simulink model "pipeline_13bit"  (R2022b)
settings: Solver=FixedStepDiscrete  StartTime=0.0  StopTime=5000*ts  FixedStep=ts  RelTol=1e-3
values from neighbouring files (symbols this model uses):
  beta = 1.01    [ADC_13bit.m]
  bits_number = 13    [ADC_13bit.m]
  C = 10e-12    (= 1e-11)    [ADC_13bit.m]
  fin = antismear(fin_pre,fs,nfft)    [ADC_13bit.m]
  Gain = 5000    [ADC_13bit.m]
  k = 1.380649e-23    [ADC_13bit.m]
  T = 300    [ADC_13bit.m]
  ts = 1/fs    (= 1)    [ADC_13bit.m]
(part 2 of 3)

== system pipeline_13bit/SHA_less_13_bit/Adder/Add6 ==
  A : Inport
  B : Inport  Port=2
  C : Inport  Port=3
  Combinatorial Logic1 : CombinatorialLogic  TruthTable=[0 0;1 0 ;1 0;0 1;1 0;0 1;0 1;1 1]
  Data Type Conversion : DataTypeConversion  OutDataTypeStr=boolean  SaturateOnIntegerOverflow=off  RndMeth=Floor
  Data Type Conversion1 : DataTypeConversion  OutDataTypeStr=double  SaturateOnIntegerOverflow=off  RndMeth=Floor
  Demux : Demux  Outputs=2
  Mux : Mux  Inputs=3
  Carry : Outport
  Sum : Outport  Port=2
  wires:
  Demux/1 -> Sum/1
  Demux/2 -> Carry/1
  Combinatorial Logic1/1 -> Data Type Conversion1/1
  Mux/1 -> Data Type Conversion/1
  A/1 -> Mux/3
  B/1 -> Mux/2
  C/1 -> Mux/1
  Data Type Conversion1/1 -> Demux/1
  Data Type Conversion/1 -> Combinatorial Logic1/1

== system pipeline_13bit/SHA_less_13_bit/Adder/Add7 ==
  A : Inport
  B : Inport  Port=2
  C : Inport  Port=3
  Combinatorial Logic1 : CombinatorialLogic  TruthTable=[0 0;1 0 ;1 0;0 1;1 0;0 1;0 1;1 1]
  Data Type Conversion : DataTypeConversion  OutDataTypeStr=boolean  SaturateOnIntegerOverflow=off  RndMeth=Floor
  Data Type Conversion1 : DataTypeConversion  OutDataTypeStr=double  SaturateOnIntegerOverflow=off  RndMeth=Floor
  Demux : Demux  Outputs=2
  Mux : Mux  Inputs=3
  Carry : Outport
  Sum : Outport  Port=2
  wires:
  Demux/1 -> Sum/1
  Demux/2 -> Carry/1
  Combinatorial Logic1/1 -> Data Type Conversion1/1
  Mux/1 -> Data Type Conversion/1
  A/1 -> Mux/3
  B/1 -> Mux/2
  C/1 -> Mux/1
  Data Type Conversion1/1 -> Demux/1
  Data Type Conversion/1 -> Combinatorial Logic1/1

== system pipeline_13bit/SHA_less_13_bit/Adder/Add8 ==
  A : Inport
  B : Inport  Port=2
  C : Inport  Port=3
  Combinatorial Logic1 : CombinatorialLogic  TruthTable=[0 0;1 0 ;1 0;0 1;1 0;0 1;0 1;1 1]
  Data Type Conversion : DataTypeConversion  OutDataTypeStr=boolean  SaturateOnIntegerOverflow=off  RndMeth=Floor
  Data Type Conversion1 : DataTypeConversion  OutDataTypeStr=double  SaturateOnIntegerOverflow=off  RndMeth=Floor
  Demux : Demux  Outputs=2
  Mux : Mux  Inputs=3
  Carry : Outport
  Sum : Outport  Port=2
  wires:
  Demux/1 -> Sum/1
  Demux/2 -> Carry/1
  Combinatorial Logic1/1 -> Data Type Conversion1/1
  Mux/1 -> Data Type Conversion/1
  A/1 -> Mux/3
  B/1 -> Mux/2
  C/1 -> Mux/1
  Data Type Conversion1/1 -> Demux/1
  Data Type Conversion/1 -> Combinatorial Logic1/1

== system pipeline_13bit/SHA_less_13_bit/Adder/Add9 ==
  A : Inport
  B : Inport  Port=2
  C : Inport  Port=3
  Combinatorial Logic1 : CombinatorialLogic  TruthTable=[0 0;1 0 ;1 0;0 1;1 0;0 1;0 1;1 1]
  Data Type Conversion : DataTypeConversion  OutDataTypeStr=boolean  SaturateOnIntegerOverflow=off  RndMeth=Floor
  Data Type Conversion1 : DataTypeConversion  OutDataTypeStr=double  SaturateOnIntegerOverflow=off  RndMeth=Floor
  Demux : Demux  Outputs=2
  Mux : Mux  Inputs=3
  Carry : Outport
  Sum : Outport  Port=2
  wires:
  Demux/1 -> Sum/1
  Demux/2 -> Carry/1
  Combinatorial Logic1/1 -> Data Type Conversion1/1
  Mux/1 -> Data Type Conversion/1
  A/1 -> Mux/3
  B/1 -> Mux/2
  C/1 -> Mux/1
  Data Type Conversion1/1 -> Demux/1
  Data Type Conversion/1 -> Combinatorial Logic1/1

== system pipeline_13bit/SHA_less_13_bit/Subsystem/stage_1p5_bit1 ==
  note: b2
  note: b1
  Vin : Inport
  Comparator 1 : Subsystem
  Comparator 2 : Subsystem
  Encoder : Subsystem
  Gain1 : Gain  Gain=2
  Gain2 : Gain
  Gain3 : Gain
  Saturation : Saturate  UpperLimit=1  LowerLimit=-1
  Sub DAC : Subsystem
  Subsystem1 : Subsystem
  Sum : Sum  Inputs=|+-
  Vref 1 : Constant  Value=-1/4
  Vref 2 : Constant  Value=1/4
  Zero-Order Hold : ZeroOrderHold  SampleTime=ts
  Residue : Outport
  D0 : Outport  Port=2
  D1 : Outport  Port=3
  wires:
  Vref 1/1 -> Comparator 1/2(Vref)
  Gain1/1 -> Sum/1
  Gain3/1 -> Sum/2
  Sum/1 -> Gain2/1
  Saturation/1 -> Zero-Order Hold/1
  Zero-Order Hold/1 -> Residue/1
  Gain2/1 -> Saturation/1
  Vref 2/1 -> Comparator 2/2(Vref)
  Comparator 2/1(Out) -> Sub DAC/2(b2), Encoder/2(b2)
  Vin/1 -> Subsystem1/1(IN)
  Comparator 1/1(Out) -> Encoder/1(b1), Sub DAC/1(b1)
  Subsystem1/1(S/H) -> Gain1/1, Comparator 1/1(Vin), Comparator 2/1(Vin)
  Sub DAC/1(Vdac) -> Gain3/1
  Encoder/1(D0) -> D0/1
  Encoder/2(D1) -> D1/1

== system pipeline_13bit/SHA_less_13_bit/Subsystem/stage_1p5_bit2 ==
  note: b2
  note: b1
  Vin : Inport
  Comparator 1 : Subsystem
  Comparator 2 : Subsystem
  Encoder : Subsystem
  Gain1 : Gain  Gain=2
  Gain2 : Gain
  Gain3 : Gain
  Saturation : Saturate  UpperLimit=1  LowerLimit=-1
  Sub DAC : Subsystem
  Subsystem1 : Subsystem
  Sum : Sum  Inputs=|+-
  Vref 1 : Constant  Value=-1/4
  Vref 2 : Constant  Value=1/4
  Zero-Order Hold : ZeroOrderHold  SampleTime=ts
  Residue : Outport
  D0 : Outport  Port=2
  D1 : Outport  Port=3
  wires:
  Vref 1/1 -> Comparator 1/2(Vref)
  Gain1/1 -> Sum/1
  Gain3/1 -> Sum/2
  Sum/1 -> Gain2/1
  Saturation/1 -> Zero-Order Hold/1
  Zero-Order Hold/1 -> Residue/1
  Gain2/1 -> Saturation/1
  Vref 2/1 -> Comparator 2/2(Vref)
  Comparator 2/1(Out) -> Sub DAC/2(b2), Encoder/2(b2)
  Vin/1 -> Subsystem1/1(IN)
  Comparator 1/1(Out) -> Encoder/1(b1), Sub DAC/1(b1)
  Subsystem1/1(S/H) -> Gain1/1, Comparator 1/1(Vin), Comparator 2/1(Vin)
  Sub DAC/1(Vdac) -> Gain3/1
  Encoder/1(D0) -> D0/1
  Encoder/2(D1) -> D1/1

== system pipeline_13bit/SHA_less_13_bit/Subsystem/stage_1p5_bit4 ==
  note: b2
  note: b1
  Vin : Inport
  Comparator 1 : Subsystem
  Comparator 2 : Subsystem
  Encoder : Subsystem
  Gain1 : Gain  Gain=2
  Gain2 : Gain
  Gain3 : Gain
  Saturation : Saturate  UpperLimit=1  LowerLimit=-1
  Sub DAC : Subsystem
  Subsystem1 : Subsystem
  Sum : Sum  Inputs=|+-
  Vref 1 : Constant  Value=-1/4
  Vref 2 : Constant  Value=1/4
  Zero-Order Hold : ZeroOrderHold  SampleTime=ts
  Residue : Outport
  D0 : Outport  Port=2
  D1 : Outport  Port=3
  wires:
  Vref 1/1 -> Comparator 1/2(Vref)
  Gain1/1 -> Sum/1
  Gain3/1 -> Sum/2
  Sum/1 -> Gain2/1
  Saturation/1 -> Zero-Order Hold/1
  Zero-Order Hold/1 -> Residue/1
  Gain2/1 -> Saturation/1
  Vref 2/1 -> Comparator 2/2(Vref)
  Comparator 2/1(Out) -> Sub DAC/2(b2), Encoder/2(b2)
  Vin/1 -> Subsystem1/1(IN)
  Comparator 1/1(Out) -> Encoder/1(b1), Sub DAC/1(b1)
  Subsystem1/1(S/H) -> Gain1/1, Comparator 1/1(Vin), Comparator 2/1(Vin)
  Sub DAC/1(Vdac) -> Gain3/1
  Encoder/1(D0) -> D0/1
  Encoder/2(D1) -> D1/1

== system pipeline_13bit/SHA_less_13_bit/Subsystem/stage_1p5_bit5 ==
  note: b2
  note: b1
  Vin : Inport
  Comparator 1 : Subsystem
  Comparator 2 : Subsystem
  Encoder : Subsystem
  Gain1 : Gain  Gain=2
  Gain2 : Gain
  Gain3 : Gain
  Saturation : Saturate  UpperLimit=1  LowerLimit=-1
  Sub DAC : Subsystem
  Subsystem1 : Subsystem
  Sum : Sum  Inputs=|+-
  Vref 1 : Constant  Value=-1/4
  Vref 2 : Constant  Value=1/4
  Zero-Order Hold : ZeroOrderHold  SampleTime=ts
  Residue : Outport
  D0 : Outport  Port=2
  D1 : Outport  Port=3
  wires:
  Vref 1/1 -> Comparator 1/2(Vref)
  Gain1/1 -> Sum/1
  Gain3/1 -> Sum/2
  Sum/1 -> Gain2/1
  Saturation/1 -> Zero-Order Hold/1
  Zero-Order Hold/1 -> Residue/1
  Gain2/1 -> Saturation/1
  Vref 2/1 -> Comparator 2/2(Vref)
  Comparator 2/1(Out) -> Sub DAC/2(b2), Encoder/2(b2)
  Vin/1 -> Subsystem1/1(IN)
  Comparator 1/1(Out) -> Encoder/1(b1), Sub DAC/1(b1)
  Subsystem1/1(S/H) -> Gain1/1, Comparator 1/1(Vin), Comparator 2/1(Vin)
  Sub DAC/1(Vdac) -> Gain3/1
  Encoder/1(D0) -> D0/1
  Encoder/2(D1) -> D1/1

== system pipeline_13bit/SHA_less_13_bit/Subsystem/stage_1p5_bit6 ==
  note: b2
  note: b1
  Vin : Inport
  Comparator 1 : Subsystem
  Comparator 2 : Subsystem
  Encoder : Subsystem
  Gain1 : Gain  Gain=2
  Gain2 : Gain
  Gain3 : Gain
  Saturation : Saturate  UpperLimit=1  LowerLimit=-1
  Sub DAC : Subsystem
  Subsystem1 : Subsystem
  Sum : Sum  Inputs=|+-
  Vref 1 : Constant  Value=-1/4
  Vref 2 : Constant  Value=1/4
  Zero-Order Hold : ZeroOrderHold  SampleTime=ts
  Residue : Outport
  D0 : Outport  Port=2
  D1 : Outport  Port=3
  wires:
  Vref 1/1 -> Comparator 1/2(Vref)
  Gain1/1 -> Sum/1
  Gain3/1 -> Sum/2
  Sum/1 -> Gain2/1
  Saturation/1 -> Zero-Order Hold/1
  Zero-Order Hold/1 -> Residue/1
  Gain2/1 -> Saturation/1
  Vref 2/1 -> Comparator 2/2(Vref)
  Comparator 2/1(Out) -> Sub DAC/2(b2), Encoder/2(b2)
  Vin/1 -> Subsystem1/1(IN)
  Comparator 1/1(Out) -> Encoder/1(b1), Sub DAC/1(b1)
  Subsystem1/1(S/H) -> Gain1/1, Comparator 1/1(Vin), Comparator 2/1(Vin)
  Sub DAC/1(Vdac) -> Gain3/1
  Encoder/1(D0) -> D0/1
  Encoder/2(D1) -> D1/1

== system pipeline_13bit/SHA_less_13_bit/Subsystem/stage_1p5_bit7 ==
  note: b2
  note: b1
  Vin : Inport
  Comparator 1 : Subsystem
  Comparator 2 : Subsystem
  Encoder : Subsystem
  Gain1 : Gain  Gain=2
  Gain2 : Gain
  Gain3 : Gain
  Saturation : Saturate  UpperLimit=1  LowerLimit=-1
  Sub DAC : Subsystem
  Subsystem1 : Subsystem
  Sum : Sum  Inputs=|+-
  Vref 1 : Constant  Value=-1/4
  Vref 2 : Constant  Value=1/4
  Zero-Order Hold : ZeroOrderHold  SampleTime=ts
  Residue : Outport
  D0 : Outport  Port=2
  D1 : Outport  Port=3
  wires:
  Vref 1/1 -> Comparator 1/2(Vref)
  Gain1/1 -> Sum/1
  Gain3/1 -> Sum/2
  Sum/1 -> Gain2/1
  Saturation/1 -> Zero-Order Hold/1
  Zero-Order Hold/1 -> Residue/1
  Gain2/1 -> Saturation/1
  Vref 2/1 -> Comparator 2/2(Vref)
  Comparator 2/1(Out) -> Sub DAC/2(b2), Encoder/2(b2)
  Vin/1 -> Subsystem1/1(IN)
  Comparator 1/1(Out) -> Encoder/1(b1), Sub DAC/1(b1)
  Subsystem1/1(S/H) -> Gain1/1, Comparator 1/1(Vin), Comparator 2/1(Vin)
  Sub DAC/1(Vdac) -> Gain3/1
  Encoder/1(D0) -> D0/1
  Encoder/2(D1) -> D1/1

== system pipeline_13bit/SHA_less_13_bit/Subsystem/stage_1p5_bit8 ==
  note: b2
  note: b1
  Vin : Inport
  Comparator 1 : Subsystem
  Comparator 2 : Subsystem
  Encoder : Subsystem
  Gain1 : Gain  Gain=2
  Gain2 : Gain
  Gain3 : Gain
  Saturation : Saturate  UpperLimit=1  LowerLimit=-1
  Sub DAC : Subsystem
  Subsystem1 : Subsystem
  Sum : Sum  Inputs=|+-
  Vref 1 : Constant  Value=-1/4
  Vref 2 : Constant  Value=1/4
  Zero-Order Hold : ZeroOrderHold  SampleTime=ts
  Residue : Outport
  D0 : Outport  Port=2
  D1 : Outport  Port=3
  wires:
  Vref 1/1 -> Comparator 1/2(Vref)
  Gain1/1 -> Sum/1
  Gain3/1 -> Sum/2
  Sum/1 -> Gain2/1
  Saturation/1 -> Zero-Order Hold/1
  Zero-Order Hold/1 -> Residue/1
  Gain2/1 -> Saturation/1
  Vref 2/1 -> Comparator 2/2(Vref)
  Comparator 2/1(Out) -> Sub DAC/2(b2), Encoder/2(b2)
  Vin/1 -> Subsystem1/1(IN)
  Comparator 1/1(Out) -> Encoder/1(b1), Sub DAC/1(b1)
  Subsystem1/1(S/H) -> Gain1/1, Comparator 1/1(Vin), Comparator 2/1(Vin)
  Sub DAC/1(Vdac) -> Gain3/1
  Encoder/1(D0) -> D0/1
  Encoder/2(D1) -> D1/1

== system pipeline_13bit/SHA_less_13_bit/Subsystem/stage_3_bit_flash ==
  Vin : Inport
  Comparator 1 : Subsystem
  Comparator 2 : Subsystem
  Comparator 3 : Subsystem
  Comparator 4 : Subsystem
  Comparator 5 : Subsystem
  Comparator 6 : Subsystem
  Comparator 7 : Subsystem
  Subsystem1 : Subsystem
  Thermometer to Binary Encoder : Subsystem
  Vref 1 : Constant  Value=-3/4
  Vref 2 : Constant  Value=-2/4
  Vref 3 : Constant  Value=-1/4
  Vref 4 : Constant  Value=0
  Vref 5 : Constant  Value=1/4
  Vref 6 : Constant  Value=2/4
  Vref 7 : Constant  Value=3/4
  Zero-Order Hold : ZeroOrderHold  SampleTime=ts
  D0 : Outport
  D1 : Outport  Port=2
  D2 : Outport  Port=3
  wires:
  Vin/1 -> Subsystem1/1(IN)
  Vref 1/1 -> Comparator 1/2(Vref)
  Thermometer to Binary Encoder/1(D0) -> D0/1
  Thermometer to Binary Encoder/2(D1) -> D1/1
  Thermometer to Binary Encoder/3(D2) -> D2/1
  Comparator 1/1(Out) -> Thermometer to Binary Encoder/1(b1)
  Vref 2/1 -> Comparator 2/2(Vref)
  Comparator 2/1(Out) -> Thermometer to Binary Encoder/2(b2)
  Vref 3/1 -> Comparator 3/2(Vref)
  Comparator 3/1(Out) -> Thermometer to Binary Encoder/3(b3)
  Vref 4/1 -> Comparator 4/2(Vref)
  Comparator 4/1(Out) -> Thermometer to Binary Encoder/4(b4)
  Vref 5/1 -> Comparator 5/2(Vref)
  Comparator 5/1(Out) -> Thermometer to Binary Encoder/5(b5)
  Vref 6/1 -> Comparator 6/2(Vref)
  Comparator 6/1(Out) -> Thermometer to Binary Encoder/6(b6)
  Vref 7/1 -> Comparator 7/2(Vref)
  Comparator 7/1(Out) -> Thermometer to Binary Encoder/7(b7)
  Zero-Order Hold/1 -> Comparator 1/1(Vin), Comparator 2/1(Vin), Comparator 3/1(Vin), Comparator 4/1(Vin), Comparator 5/1(Vin), Comparator 6/1(Vin), Comparator 7/1(Vin)
  Subsystem1/1(S/H) -> Zero-Order Hold/1

== system pipeline_13bit/SHA_less_13_bit/Subsystem/stage_3p5_bit ==
  Vin : Inport
  Encoder : Subsystem
  Gain1 : Gain  Gain=8
  Gain2 : Gain
  Gain3 : Gain
  Saturation : Saturate  UpperLimit=1000  LowerLimit=-1
  Sub ADC : Subsystem
      settings: PortSchema="{\"entries\":[{\"content\":{\"sides\":[{\"content\":{\"connectorIds\":[]},\"type\":\"ConnectorPlacement.EquallySpacedRectSide\",\"uuid\":\"1d580c1c-4142-4e48-88a4-e1fd0f0e227e\"},{\"content\":{\"connectorIds\":[\"Out1\",\"Out2\",\"Out3\",\"Out4\",\"Out5\",\"Out6\",\"Out7\",\"Out8\",\"Out9\",\"Out10\",\"Out11\",\"Out12\",\"Out13\",\"Out14\"],\"side\":\"RIGHT\"},\"type\":\"ConnectorPlacement.EquallySpacedRectSide\",\"uuid\":\"3d052ec1-94f1-45dc-924d-acfea8c79606\"},{\"content\":{\"connectorIds\":[\"In1\"],\"side\":\"TOP\"},\"type\":\"ConnectorPlacement.EquallySpacedRectSide\",\"uuid\":\"20df264a-1a70-4325-b402-c0ed20a64841\"}]},\"type\":\"ConnectorPlacement.EquallySpacedConnector\",\"uuid\":\"3e6ddb48-a356-47ca-8914-cd3660926421\"}],\"packageUris\":[\"http://schema.mathworks.com/mf0/Connector/R2020b\"],\"version\":\"1.0\"}"
  Sub DAC : Subsystem
      settings: PortSchema="{\"entries\":[{\"content\":{\"sides\":[{\"content\":{\"connectorIds\":[\"In1\",\"In2\",\"In3\",\"In4\",\"In5\",\"In6\",\"In7\",\"In8\",\"In9\",\"In10\",\"In11\",\"In12\",\"In13\",\"In14\"]},\"type\":\"ConnectorPlacement.EquallySpacedRectSide\",\"uuid\":\"d439bcb5-51fb-4878-814b-2d8ac36d8f53\"},{\"content\":{\"connectorIds\":[],\"side\":\"RIGHT\"},\"type\":\"ConnectorPlacement.EquallySpacedRectSide\",\"uuid\":\"a7e6c2a3-22c0-4c5a-aa3b-05f7415ac298\"},{\"content\":{\"connectorIds\":[\"Out1\"],\"side\":\"TOP\"},\"type\":\"ConnectorPlacement.EquallySpacedRectSide\",\"uuid\":\"e0a2b774-5ae1-46ea-b76d-1a34ecfd289b\"}]},\"type\":\"ConnectorPlacement.EquallySpacedConnector\",\"uuid\":\"f57b1e36-985f-4826-993f-0988339ac824\"}],\"packageUris\":[\"http://schema.mathworks.com/mf0/Connector/R2020b\"],\"version\":\"1.0\"}"
  Subsystem1 : Subsystem
  Sum : Sum  Inputs=|+-
  Zero-Order Hold : ZeroOrderHold  SampleTime=ts
  Residue : Outport
  D0 : Outport  Port=2
  D1 : Outport  Port=3
  D2 : Outport  Port=4
  D3 : Outport  Port=5
  wires:
  Gain1/1 -> Sum/1
  Gain3/1 -> Sum/2
  Sum/1 -> Gain2/1
  Saturation/1 -> Zero-Order Hold/1
  Gain2/1 -> Saturation/1
  Encoder/1(D0) -> D0/1
  Encoder/3(D2) -> D2/1
  Encoder/2(D1) -> D1/1
  Vin/1 -> Subsystem1/1(IN)
  Encoder/4(D3) -> D3/1
  Zero-Order Hold/1 -> Residue/1
  Subsystem1/1(S/H) -> Gain1/1, Sub ADC/1(Vin)
  Sub ADC/1(b1) -> Encoder/1(b1), Sub DAC/1(b1)
  Sub ADC/2(b2) -> Encoder/2(b2), Sub DAC/2(b2)
  Sub ADC/3(b3) -> Sub DAC/3(b3), Encoder/3(b3)
  Sub ADC/4(b4) -> Sub DAC/4(b4), Encoder/4(b4)
  Sub ADC/5(b5) -> Sub DAC/5(b5), Encoder/5(b5)
  Sub ADC/6(b6) -> Encoder/6(b6), Sub DAC/6(b6)
  Sub ADC/7(b7) -> Encoder/7(b7), Sub DAC/7(b7)
  Sub ADC/8(b8) -> Encoder/8(b8), Sub DAC/8(b8)
  Sub ADC/9(b9) -> Encoder/9(b9), Sub DAC/9(b9)
  Sub ADC/10(b10) -> Encoder/10(b10), Sub DAC/10(b10)
  Sub ADC/11(b11) -> Sub DAC/11(b11), Encoder/11(b11)
  Sub ADC/12(b12) -> Sub DAC/12(b12), Encoder/12(b12)
  Sub ADC/13(b13) -> Encoder/13(b13), Sub DAC/13(b13)
  Sub ADC/14(b14) -> Encoder/14(b14), Sub DAC/14(b14)
  Sub DAC/1(Vdac) -> Gain3/1

== system pipeline_13bit/13_bit/Subsystem/Subsystem/Clock Jitter ==
  IN : Inport
  Derivative : Derivative
  Product : Product
  Random Number : RandomNumber  SampleTime=ts
  Sum : Sum
  Zero-Order Hold2 : ZeroOrderHold  SampleTime=ts
  Zero-Order Hold3 : ZeroOrderHold  SampleTime=ts
  delta : Gain  Gain=0.02
  Clock : Outport
  wires:
  IN/1 -> Derivative/1, Sum/1
  Product/1 -> Sum/2
  Derivative/1 -> Product/1
  Zero-Order Hold2/1 -> delta/1
  Sum/1 -> Zero-Order Hold3/1
  delta/1 -> Product/2
  Zero-Order Hold3/1 -> Clock/1
  Random Number/1 -> Zero-Order Hold2/1

== system pipeline_13bit/13_bit/Subsystem/Subsystem/GainError ==
  Constant : Constant  Value=Gain  SampleTime=-1
  Constant1 : Constant  Value=beta  SampleTime=-1
  MATLAB Function : MATLAB Function  TreatAsAtomicUnit=on
  Product1 : Product
  GainError : Outport
  wires:
  Constant/1 -> Product1/1
  Constant1/1 -> Product1/2
  Product1/1 -> MATLAB Function/1(u)
  MATLAB Function/1(y) -> GainError/1

== system pipeline_13bit/13_bit/Subsystem/Subsystem/KT//C Noise ==
  Constant : Constant  Value=sqrt((k*T/C))  SampleTime=-1
  Product1 : Product
  Random Number : RandomNumber  SampleTime=ts
  Zero-Order Hold2 : ZeroOrderHold  SampleTime=ts
  KT/C Noise : Outport
  wires:
  Random Number/1 -> Zero-Order Hold2/1
  Product1/1 -> KT/C Noise/1
  Zero-Order Hold2/1 -> Product1/2
  Constant/1 -> Product1/1

== system pipeline_13bit/13_bit/Subsystem/Subsystem/Subsystem1 ==
  Gain1 : Gain  Gain=0.02
  Random Number : RandomNumber  SampleTime=ts
  Zero-Order Hold2 : ZeroOrderHold  SampleTime=ts
  Op Noise : Outport
  wires:
  Random Number/1 -> Zero-Order Hold2/1
  Gain1/1 -> Op Noise/1
  Zero-Order Hold2/1 -> Gain1/1

== system pipeline_13bit/13_bit/Subsystem/stage_1p5_bit1/Comparator 1 ==
  Vin : Inport
  Vref : Inport  Port=2
  Output 1 or 0 : Relay  OnSwitchValue=0  OffSwitchValue=0
  Sum : Sum  Inputs=|+-
  Out : Outport
  wires:
  Sum/1 -> Output 1 or 0/1
  Vin/1 -> Sum/1
  Output 1 or 0/1 -> Out/1
  Vref/1 -> Sum/2

== system pipeline_13bit/13_bit/Subsystem/stage_1p5_bit1/Comparator 2 ==
  Vin : Inport
  Vref : Inport  Port=2
  Output 1 or 0 : Relay  OnSwitchValue=0  OffSwitchValue=0
  Sum : Sum  Inputs=|+-
  Out : Outport
  wires:
  Sum/1 -> Output 1 or 0/1
  Vin/1 -> Sum/1
  Output 1 or 0/1 -> Out/1
  Vref/1 -> Sum/2

== system pipeline_13bit/13_bit/Subsystem/stage_1p5_bit1/Encoder ==
  b1 : Inport
  b2 : Inport  Port=2
  " " : DataTypeConversion  OutDataTypeStr=double  SaturateOnIntegerOverflow=off  RndMeth=Floor
  NOR : Logic  Operator=NOR  AllPortsSameDT=off  OutDataTypeStr=boolean
  NOT : Logic  Operator=NOT  AllPortsSameDT=off  OutDataTypeStr=boolean
  D0 : Outport
  D1 : Outport  Port=2
  wires:
  b2/1 -> NOR/2, D1/1
  NOR/1 -> " "/1
  " "/1 -> D0/1
  NOT/1 -> NOR/1
  b1/1 -> NOT/1

== system pipeline_13bit/13_bit/Subsystem/stage_1p5_bit1/Sub DAC ==
  b1 : Inport
  b2 : Inport  Port=2
  NOT : Logic  Operator=NOT  AllPortsSameDT=off  OutDataTypeStr=boolean
  Subtract : Sum  Inputs=-+
  Vdac : Outport
  wires:
  b2/1 -> Subtract/2
  b1/1 -> NOT/1
  Subtract/1 -> Vdac/1
  NOT/1 -> Subtract/1

== system pipeline_13bit/13_bit/Subsystem/stage_1p5_bit1/Subsystem1 ==
  IN : Inport
  Clock Jitter : Subsystem  Description=Jitter
  Gain : Gain
  Saturation : Saturate  UpperLimit=1000  LowerLimit=-1
  Zero-Order Hold1 : ZeroOrderHold  SampleTime=ts
  S/H : Outport
  wires:
  Zero-Order Hold1/1 -> S/H/1
  Saturation/1 -> Zero-Order Hold1/1
  IN/1 -> Clock Jitter/1(IN)
  Clock Jitter/1(Clock) -> Gain/1
  Gain/1 -> Saturation/1

== system pipeline_13bit/13_bit/Subsystem/stage_1p5_bit2/Comparator 1 ==
  Vin : Inport
  Vref : Inport  Port=2
  Output 1 or 0 : Relay  OnSwitchValue=0  OffSwitchValue=0
  Sum : Sum  Inputs=|+-
  Out : Outport
  wires:
  Sum/1 -> Output 1 or 0/1
  Vin/1 -> Sum/1
  Output 1 or 0/1 -> Out/1
  Vref/1 -> Sum/2

== system pipeline_13bit/13_bit/Subsystem/stage_1p5_bit2/Comparator 2 ==
  Vin : Inport
  Vref : Inport  Port=2
  Output 1 or 0 : Relay  OnSwitchValue=0  OffSwitchValue=0
  Sum : Sum  Inputs=|+-
  Out : Outport
  wires:
  Sum/1 -> Output 1 or 0/1
  Vin/1 -> Sum/1
  Output 1 or 0/1 -> Out/1
  Vref/1 -> Sum/2

== system pipeline_13bit/13_bit/Subsystem/stage_1p5_bit2/Encoder ==
  b1 : Inport
  b2 : Inport  Port=2
  " " : DataTypeConversion  OutDataTypeStr=double  SaturateOnIntegerOverflow=off  RndMeth=Floor
  NOR : Logic  Operator=NOR  AllPortsSameDT=off  OutDataTypeStr=boolean
  NOT : Logic  Operator=NOT  AllPortsSameDT=off  OutDataTypeStr=boolean
  D0 : Outport
  D1 : Outport  Port=2
  wires:
  b2/1 -> NOR/2, D1/1
  NOR/1 -> " "/1
  " "/1 -> D0/1
  NOT/1 -> NOR/1
  b1/1 -> NOT/1

== system pipeline_13bit/13_bit/Subsystem/stage_1p5_bit2/Sub DAC ==
  b1 : Inport
  b2 : Inport  Port=2
  NOT : Logic  Operator=NOT  AllPortsSameDT=off  OutDataTypeStr=boolean
  Subtract : Sum  Inputs=-+
  Vdac : Outport
  wires:
  b2/1 -> Subtract/2
  b1/1 -> NOT/1
  Subtract/1 -> Vdac/1
  NOT/1 -> Subtract/1

== system pipeline_13bit/13_bit/Subsystem/stage_1p5_bit2/Subsystem1 ==
  IN : Inport
  Clock Jitter : Subsystem  Description=Jitter
  Gain : Gain
  Saturation : Saturate  UpperLimit=1000  LowerLimit=-1
  Zero-Order Hold1 : ZeroOrderHold  SampleTime=ts
  S/H : Outport
  wires:
  Zero-Order Hold1/1 -> S/H/1
  Saturation/1 -> Zero-Order Hold1/1
  IN/1 -> Clock Jitter/1(IN)
  Clock Jitter/1(Clock) -> Gain/1
  Gain/1 -> Saturation/1

== system pipeline_13bit/13_bit/Subsystem/stage_1p5_bit4/Comparator 1 ==
  Vin : Inport
  Vref : Inport  Port=2
  Output 1 or 0 : Relay  OnSwitchValue=0  OffSwitchValue=0
  Sum : Sum  Inputs=|+-
  Out : Outport
  wires:
  Sum/1 -> Output 1 or 0/1
  Vin/1 -> Sum/1
  Output 1 or 0/1 -> Out/1
  Vref/1 -> Sum/2

== system pipeline_13bit/13_bit/Subsystem/stage_1p5_bit4/Comparator 2 ==
  Vin : Inport
  Vref : Inport  Port=2
  Output 1 or 0 : Relay  OnSwitchValue=0  OffSwitchValue=0
  Sum : Sum  Inputs=|+-
  Out : Outport
  wires:
  Sum/1 -> Output 1 or 0/1
  Vin/1 -> Sum/1
  Output 1 or 0/1 -> Out/1
  Vref/1 -> Sum/2

== system pipeline_13bit/13_bit/Subsystem/stage_1p5_bit4/Encoder ==
  b1 : Inport
  b2 : Inport  Port=2
  " " : DataTypeConversion  OutDataTypeStr=double  SaturateOnIntegerOverflow=off  RndMeth=Floor
  NOR : Logic  Operator=NOR  AllPortsSameDT=off  OutDataTypeStr=boolean
  NOT : Logic  Operator=NOT  AllPortsSameDT=off  OutDataTypeStr=boolean
  D0 : Outport
  D1 : Outport  Port=2
  wires:
  b2/1 -> NOR/2, D1/1
  NOR/1 -> " "/1
  " "/1 -> D0/1
  NOT/1 -> NOR/1
  b1/1 -> NOT/1

== system pipeline_13bit/13_bit/Subsystem/stage_1p5_bit4/Sub DAC ==
  b1 : Inport
  b2 : Inport  Port=2
  NOT : Logic  Operator=NOT  AllPortsSameDT=off  OutDataTypeStr=boolean
  Subtract : Sum  Inputs=-+
  Vdac : Outport
  wires:
  b2/1 -> Subtract/2
  b1/1 -> NOT/1
  Subtract/1 -> Vdac/1
  NOT/1 -> Subtract/1

== system pipeline_13bit/13_bit/Subsystem/stage_1p5_bit4/Subsystem1 ==
  IN : Inport
  Clock Jitter : Subsystem  Description=Jitter
  Gain : Gain
  Saturation : Saturate  UpperLimit=1000  LowerLimit=-1
  Zero-Order Hold1 : ZeroOrderHold  SampleTime=ts
  S/H : Outport
  wires:
  Zero-Order Hold1/1 -> S/H/1
  Saturation/1 -> Zero-Order Hold1/1
  IN/1 -> Clock Jitter/1(IN)
  Clock Jitter/1(Clock) -> Gain/1
  Gain/1 -> Saturation/1

== system pipeline_13bit/13_bit/Subsystem/stage_1p5_bit5/Comparator 1 ==
  Vin : Inport
  Vref : Inport  Port=2
  Output 1 or 0 : Relay  OnSwitchValue=0  OffSwitchValue=0
  Sum : Sum  Inputs=|+-
  Out : Outport
  wires:
  Sum/1 -> Output 1 or 0/1
  Vin/1 -> Sum/1
  Output 1 or 0/1 -> Out/1
  Vref/1 -> Sum/2

== system pipeline_13bit/13_bit/Subsystem/stage_1p5_bit5/Comparator 2 ==
  Vin : Inport
  Vref : Inport  Port=2
  Output 1 or 0 : Relay  OnSwitchValue=0  OffSwitchValue=0
  Sum : Sum  Inputs=|+-
  Out : Outport
  wires:
  Sum/1 -> Output 1 or 0/1
  Vin/1 -> Sum/1
  Output 1 or 0/1 -> Out/1
  Vref/1 -> Sum/2

== system pipeline_13bit/13_bit/Subsystem/stage_1p5_bit5/Encoder ==
  b1 : Inport
  b2 : Inport  Port=2
  " " : DataTypeConversion  OutDataTypeStr=double  SaturateOnIntegerOverflow=off  RndMeth=Floor
  NOR : Logic  Operator=NOR  AllPortsSameDT=off  OutDataTypeStr=boolean
  NOT : Logic  Operator=NOT  AllPortsSameDT=off  OutDataTypeStr=boolean
  D0 : Outport
  D1 : Outport  Port=2
  wires:
  b2/1 -> NOR/2, D1/1
  NOR/1 -> " "/1
  " "/1 -> D0/1
  NOT/1 -> NOR/1
  b1/1 -> NOT/1

== system pipeline_13bit/13_bit/Subsystem/stage_1p5_bit5/Sub DAC ==
  b1 : Inport
  b2 : Inport  Port=2
  NOT : Logic  Operator=NOT  AllPortsSameDT=off  OutDataTypeStr=boolean
  Subtract : Sum  Inputs=-+
  Vdac : Outport
  wires:
  b2/1 -> Subtract/2
  b1/1 -> NOT/1
  Subtract/1 -> Vdac/1
  NOT/1 -> Subtract/1

== system pipeline_13bit/13_bit/Subsystem/stage_1p5_bit5/Subsystem1 ==
  IN : Inport
  Clock Jitter : Subsystem  Description=Jitter
  Gain : Gain
  Saturation : Saturate  UpperLimit=1000  LowerLimit=-1
  Zero-Order Hold1 : ZeroOrderHold  SampleTime=ts
  S/H : Outport
  wires:
  Zero-Order Hold1/1 -> S/H/1
  Saturation/1 -> Zero-Order Hold1/1
  IN/1 -> Clock Jitter/1(IN)
  Clock Jitter/1(Clock) -> Gain/1
  Gain/1 -> Saturation/1

== system pipeline_13bit/13_bit/Subsystem/stage_1p5_bit6/Comparator 1 ==
  Vin : Inport
  Vref : Inport  Port=2
  Output 1 or 0 : Relay  OnSwitchValue=0  OffSwitchValue=0
  Sum : Sum  Inputs=|+-
  Out : Outport
  wires:
  Sum/1 -> Output 1 or 0/1
  Vin/1 -> Sum/1
  Output 1 or 0/1 -> Out/1
  Vref/1 -> Sum/2

== system pipeline_13bit/13_bit/Subsystem/stage_1p5_bit6/Comparator 2 ==
  Vin : Inport
  Vref : Inport  Port=2
  Output 1 or 0 : Relay  OnSwitchValue=0  OffSwitchValue=0
  Sum : Sum  Inputs=|+-
  Out : Outport
  wires:
  Sum/1 -> Output 1 or 0/1
  Vin/1 -> Sum/1
  Output 1 or 0/1 -> Out/1
  Vref/1 -> Sum/2

== system pipeline_13bit/13_bit/Subsystem/stage_1p5_bit6/Encoder ==
  b1 : Inport
  b2 : Inport  Port=2
  " " : DataTypeConversion  OutDataTypeStr=double  SaturateOnIntegerOverflow=off  RndMeth=Floor
  NOR : Logic  Operator=NOR  AllPortsSameDT=off  OutDataTypeStr=boolean
  NOT : Logic  Operator=NOT  AllPortsSameDT=off  OutDataTypeStr=boolean
  D0 : Outport
  D1 : Outport  Port=2
  wires:
  b2/1 -> NOR/2, D1/1
  NOR/1 -> " "/1
  " "/1 -> D0/1
  NOT/1 -> NOR/1
  b1/1 -> NOT/1

== system pipeline_13bit/13_bit/Subsystem/stage_1p5_bit6/Sub DAC ==
  b1 : Inport
  b2 : Inport  Port=2
  NOT : Logic  Operator=NOT  AllPortsSameDT=off  OutDataTypeStr=boolean
  Subtract : Sum  Inputs=-+
  Vdac : Outport
  wires:
  b2/1 -> Subtract/2
  b1/1 -> NOT/1
  Subtract/1 -> Vdac/1
  NOT/1 -> Subtract/1

== system pipeline_13bit/13_bit/Subsystem/stage_1p5_bit6/Subsystem1 ==
  IN : Inport
  Clock Jitter : Subsystem  Description=Jitter
  Gain : Gain
  Saturation : Saturate  UpperLimit=1000  LowerLimit=-1
  Zero-Order Hold1 : ZeroOrderHold  SampleTime=ts
  S/H : Outport
  wires:
  Zero-Order Hold1/1 -> S/H/1
  Saturation/1 -> Zero-Order Hold1/1
  IN/1 -> Clock Jitter/1(IN)
  Clock Jitter/1(Clock) -> Gain/1
  Gain/1 -> Saturation/1

== system pipeline_13bit/13_bit/Subsystem/stage_1p5_bit7/Comparator 1 ==
  Vin : Inport
  Vref : Inport  Port=2
  Output 1 or 0 : Relay  OnSwitchValue=0  OffSwitchValue=0
  Sum : Sum  Inputs=|+-
  Out : Outport
  wires:
  Sum/1 -> Output 1 or 0/1
  Vin/1 -> Sum/1
  Output 1 or 0/1 -> Out/1
  Vref/1 -> Sum/2

== system pipeline_13bit/13_bit/Subsystem/stage_1p5_bit7/Comparator 2 ==
  Vin : Inport
  Vref : Inport  Port=2
  Output 1 or 0 : Relay  OnSwitchValue=0  OffSwitchValue=0
  Sum : Sum  Inputs=|+-
  Out : Outport
  wires:
  Sum/1 -> Output 1 or 0/1
  Vin/1 -> Sum/1
  Output 1 or 0/1 -> Out/1
  Vref/1 -> Sum/2

== system pipeline_13bit/13_bit/Subsystem/stage_1p5_bit7/Encoder ==
  b1 : Inport
  b2 : Inport  Port=2
  " " : DataTypeConversion  OutDataTypeStr=double  SaturateOnIntegerOverflow=off  RndMeth=Floor
  NOR : Logic  Operator=NOR  AllPortsSameDT=off  OutDataTypeStr=boolean
  NOT : Logic  Operator=NOT  AllPortsSameDT=off  OutDataTypeStr=boolean
  D0 : Outport
  D1 : Outport  Port=2
  wires:
  b2/1 -> NOR/2, D1/1
  NOR/1 -> " "/1
  " "/1 -> D0/1
  NOT/1 -> NOR/1
  b1/1 -> NOT/1

== system pipeline_13bit/13_bit/Subsystem/stage_1p5_bit7/Sub DAC ==
  b1 : Inport
  b2 : Inport  Port=2
  NOT : Logic  Operator=NOT  AllPortsSameDT=off  OutDataTypeStr=boolean
  Subtract : Sum  Inputs=-+
  Vdac : Outport
  wires:
  b2/1 -> Subtract/2
  b1/1 -> NOT/1
  Subtract/1 -> Vdac/1
  NOT/1 -> Subtract/1

== system pipeline_13bit/13_bit/Subsystem/stage_1p5_bit7/Subsystem1 ==
  IN : Inport
  Clock Jitter : Subsystem  Description=Jitter
  Gain : Gain
  Saturation : Saturate  UpperLimit=1000  LowerLimit=-1
  Zero-Order Hold1 : ZeroOrderHold  SampleTime=ts
  S/H : Outport
  wires:
  Zero-Order Hold1/1 -> S/H/1
  Saturation/1 -> Zero-Order Hold1/1
  IN/1 -> Clock Jitter/1(IN)
  Clock Jitter/1(Clock) -> Gain/1
  Gain/1 -> Saturation/1

== system pipeline_13bit/13_bit/Subsystem/stage_1p5_bit8/Comparator 1 ==
  Vin : Inport
  Vref : Inport  Port=2
  Output 1 or 0 : Relay  OnSwitchValue=0  OffSwitchValue=0
  Sum : Sum  Inputs=|+-
  Out : Outport
  wires:
  Sum/1 -> Output 1 or 0/1
  Vin/1 -> Sum/1
  Output 1 or 0/1 -> Out/1
  Vref/1 -> Sum/2

== system pipeline_13bit/13_bit/Subsystem/stage_1p5_bit8/Comparator 2 ==
  Vin : Inport
  Vref : Inport  Port=2
  Output 1 or 0 : Relay  OnSwitchValue=0  OffSwitchValue=0
  Sum : Sum  Inputs=|+-
  Out : Outport
  wires:
  Sum/1 -> Output 1 or 0/1
  Vin/1 -> Sum/1
  Output 1 or 0/1 -> Out/1
  Vref/1 -> Sum/2

== system pipeline_13bit/13_bit/Subsystem/stage_1p5_bit8/Encoder ==
  b1 : Inport
  b2 : Inport  Port=2
  " " : DataTypeConversion  OutDataTypeStr=double  SaturateOnIntegerOverflow=off  RndMeth=Floor
  NOR : Logic  Operator=NOR  AllPortsSameDT=off  OutDataTypeStr=boolean
  NOT : Logic  Operator=NOT  AllPortsSameDT=off  OutDataTypeStr=boolean
  D0 : Outport
  D1 : Outport  Port=2
  wires:
  b2/1 -> NOR/2, D1/1
  NOR/1 -> " "/1
  " "/1 -> D0/1
  NOT/1 -> NOR/1
  b1/1 -> NOT/1

== system pipeline_13bit/13_bit/Subsystem/stage_1p5_bit8/Sub DAC ==
  b1 : Inport
  b2 : Inport  Port=2
  NOT : Logic  Operator=NOT  AllPortsSameDT=off  OutDataTypeStr=boolean
  Subtract : Sum  Inputs=-+
  Vdac : Outport
  wires:
  b2/1 -> Subtract/2
  b1/1 -> NOT/1
  Subtract/1 -> Vdac/1
  NOT/1 -> Subtract/1

== system pipeline_13bit/13_bit/Subsystem/stage_1p5_bit8/Subsystem1 ==
  IN : Inport
  Clock Jitter : Subsystem  Description=Jitter
  Gain : Gain
  Saturation : Saturate  UpperLimit=1000  LowerLimit=-1
  Zero-Order Hold1 : ZeroOrderHold  SampleTime=ts
  S/H : Outport
  wires:
  Zero-Order Hold1/1 -> S/H/1
  Saturation/1 -> Zero-Order Hold1/1
  IN/1 -> Clock Jitter/1(IN)
  Clock Jitter/1(Clock) -> Gain/1
  Gain/1 -> Saturation/1

== system pipeline_13bit/13_bit/Subsystem/stage_3_bit_flash/Comparator 1 ==
  Vin : Inport
  Vref : Inport  Port=2
  Output 1 or 0 : Relay  OnSwitchValue=0  OffSwitchValue=0
  Sum : Sum  Inputs=|+-
  Out : Outport
  wires:
  Sum/1 -> Output 1 or 0/1
  Vin/1 -> Sum/1
  Output 1 or 0/1 -> Out/1
  Vref/1 -> Sum/2

== system pipeline_13bit/13_bit/Subsystem/stage_3_bit_flash/Comparator 2 ==
  Vin : Inport
  Vref : Inport  Port=2
  Output 1 or 0 : Relay  OnSwitchValue=0  OffSwitchValue=0
  Sum : Sum  Inputs=|+-
  Out : Outport
  wires:
  Sum/1 -> Output 1 or 0/1
  Vin/1 -> Sum/1
  Output 1 or 0/1 -> Out/1
  Vref/1 -> Sum/2

== system pipeline_13bit/13_bit/Subsystem/stage_3_bit_flash/Comparator 3 ==
  Vin : Inport
  Vref : Inport  Port=2
  Output 1 or 0 : Relay  OnSwitchValue=0  OffSwitchValue=0
  Sum : Sum  Inputs=|+-
  Out : Outport
  wires:
  Sum/1 -> Output 1 or 0/1
  Vin/1 -> Sum/1
  Output 1 or 0/1 -> Out/1
  Vref/1 -> Sum/2

== system pipeline_13bit/13_bit/Subsystem/stage_3_bit_flash/Comparator 4 ==
  Vin : Inport
  Vref : Inport  Port=2
  Output 1 or 0 : Relay  OnSwitchValue=0  OffSwitchValue=0
  Sum : Sum  Inputs=|+-
  Out : Outport
  wires:
  Sum/1 -> Output 1 or 0/1
  Vin/1 -> Sum/1
  Output 1 or 0/1 -> Out/1
  Vref/1 -> Sum/2

== system pipeline_13bit/13_bit/Subsystem/stage_3_bit_flash/Comparator 5 ==
  Vin : Inport
  Vref : Inport  Port=2
  Output 1 or 0 : Relay  OnSwitchValue=0  OffSwitchValue=0
  Sum : Sum  Inputs=|+-
  Out : Outport
  wires:
  Sum/1 -> Output 1 or 0/1
  Vin/1 -> Sum/1
  Output 1 or 0/1 -> Out/1
  Vref/1 -> Sum/2

== system pipeline_13bit/13_bit/Subsystem/stage_3_bit_flash/Comparator 6 ==
  Vin : Inport
  Vref : Inport  Port=2
  Output 1 or 0 : Relay  OnSwitchValue=0  OffSwitchValue=0
  Sum : Sum  Inputs=|+-
  Out : Outport
  wires:
  Sum/1 -> Output 1 or 0/1
  Vin/1 -> Sum/1
  Output 1 or 0/1 -> Out/1
  Vref/1 -> Sum/2

== system pipeline_13bit/13_bit/Subsystem/stage_3_bit_flash/Comparator 7 ==
  Vin : Inport
  Vref : Inport  Port=2
  Output 1 or 0 : Relay  OnSwitchValue=0  OffSwitchValue=0
  Sum : Sum  Inputs=|+-
  Out : Outport
  wires:
  Sum/1 -> Output 1 or 0/1
  Vin/1 -> Sum/1
  Output 1 or 0/1 -> Out/1
  Vref/1 -> Sum/2

== system pipeline_13bit/13_bit/Subsystem/stage_3_bit_flash/Subsystem1 ==
  IN : Inport
  Clock Jitter : Subsystem  Description=Jitter
  Gain : Gain
  Saturation : Saturate  UpperLimit=1000  LowerLimit=-1
  Zero-Order Hold1 : ZeroOrderHold  SampleTime=ts
  S/H : Outport
  wires:
  Zero-Order Hold1/1 -> S/H/1
  Saturation/1 -> Zero-Order Hold1/1
  IN/1 -> Clock Jitter/1(IN)
  Clock Jitter/1(Clock) -> Gain/1
  Gain/1 -> Saturation/1

== system pipeline_13bit/13_bit/Subsystem/stage_3_bit_flash/Thermometer to Binary Encoder ==
  b1 : Inport
  b2 : Inport  Port=2
  b3 : Inport  Port=3
  b4 : Inport  Port=4
  b5 : Inport  Port=5
  b6 : Inport  Port=6
  b7 : Inport  Port=7
  and{,1..3} (4 alike) : Logic  AllPortsSameDT=off  OutDataTypeStr=boolean
  int1 : DataTypeConversion  OutDataTypeStr=double  SaturateOnIntegerOverflow=off  RndMeth=Floor
  int2 : DataTypeConversion  OutDataTypeStr=double  SaturateOnIntegerOverflow=off  RndMeth=Floor
  int3 : DataTypeConversion  OutDataTypeStr=double  SaturateOnIntegerOverflow=off  RndMeth=Floor
  not : Logic  Operator=NOT  AllPortsSameDT=off  OutDataTypeStr=boolean
  not1 : Logic  Operator=NOT  AllPortsSameDT=off  OutDataTypeStr=boolean
  not2 : Logic  Operator=NOT  AllPortsSameDT=off  OutDataTypeStr=boolean
  or : Logic  Operator=OR  AllPortsSameDT=off  OutDataTypeStr=boolean
  or1 : Logic  Operator=OR  Inputs=4  AllPortsSameDT=off  OutDataTypeStr=boolean
  D0 : Outport
  D1 : Outport  Port=2
  D2 : Outport  Port=3
  wires:
  b4/1 -> not/1, int1/1
  not/1 -> and/2, and2/1
  b2/1 -> and/1, not1/1
  b6/1 -> or/2, not2/1
  and/1 -> or/1
  or/1 -> int2/1
  or1/1 -> int3/1
  b1/1 -> and1/1
  not1/1 -> and1/2
  and1/1 -> or1/1
  b3/1 -> and2/2
  and2/1 -> or1/2
  b7/1 -> or1/4
  not2/1 -> and3/2
  b5/1 -> and3/1
  int2/1 -> D1/1
  int3/1 -> D0/1
  and3/1 -> or1/3
  int1/1 -> D2/1

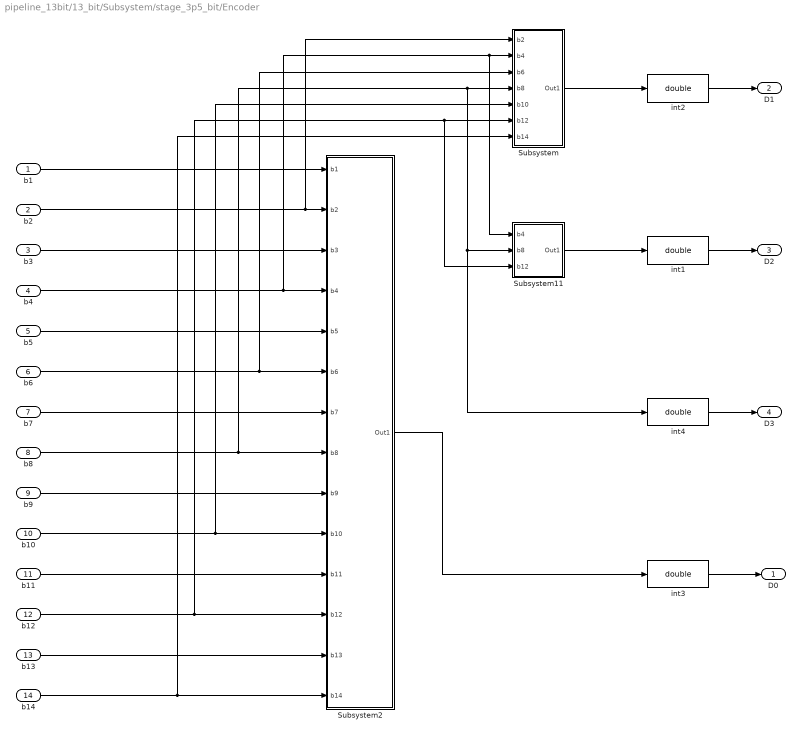
== system pipeline_13bit/13_bit/Subsystem/stage_3p5_bit/Encoder ==
  b1 : Inport
  b2 : Inport  Port=2
  b3 : Inport  Port=3
  b4 : Inport  Port=4
  b5 : Inport  Port=5
  b6 : Inport  Port=6
  b7 : Inport  Port=7
  b8 : Inport  Port=8
  b9 : Inport  Port=9
  b10 : Inport  Port=10
  b11 : Inport  Port=11
  b12 : Inport  Port=12
  b13 : Inport  Port=13
  b14 : Inport  Port=14
  Subsystem : Subsystem
  Subsystem11 : Subsystem
  Subsystem2 : Subsystem
  int{1..4} (4 alike) : DataTypeConversion  OutDataTypeStr=double  SaturateOnIntegerOverflow=off  RndMeth=Floor
  D0 : Outport
  D1 : Outport  Port=2
  D2 : Outport  Port=3
  D3 : Outport  Port=4
  wires:
  int2/1 -> D1/1
  int3/1 -> D0/1
  int1/1 -> D2/1
  int4/1 -> D3/1
  Subsystem11/1(Out1) -> int1/1
  Subsystem/1(Out1) -> int2/1
  Subsystem2/1(Out1) -> int3/1
  b1/1 -> Subsystem2/1(b1)
  b2/1 -> Subsystem/1(b2), Subsystem2/2(b2)
  b3/1 -> Subsystem2/3(b3)
  b4/1 -> Subsystem11/1(b4), Subsystem/2(b4), Subsystem2/4(b4)
  b5/1 -> Subsystem2/5(b5)
  b7/1 -> Subsystem2/7(b7)
  b8/1 -> Subsystem11/2(b8), int4/1, Subsystem/4(b8), Subsystem2/8(b8)
  b9/1 -> Subsystem2/9(b9)
  b10/1 -> Subsystem/5(b10), Subsystem2/10(b10)
  b11/1 -> Subsystem2/11(b11)
  b12/1 -> Subsystem11/3(b12), Subsystem/6(b12), Subsystem2/12(b12)
  b13/1 -> Subsystem2/13(b13)
  b14/1 -> Subsystem/7(b14), Subsystem2/14(b14)
  b6/1 -> Subsystem/3(b6), Subsystem2/6(b6)

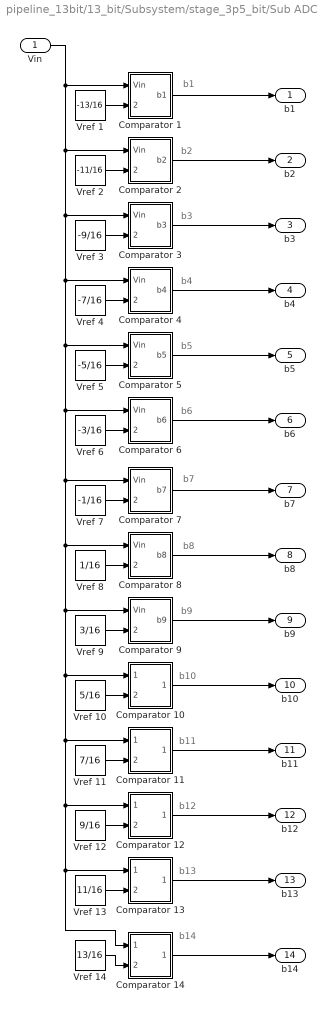
== system pipeline_13bit/13_bit/Subsystem/stage_3p5_bit/Sub ADC ==
  note: b2
  note: b1
  note: b3
  note: b4
  note: b5
  note: b6
  note: b10
  note: b11
  note: b9
  note: b12
  note: b8
  note: b7
  note: b14
  note: b13
  Vin : Inport
  Comparator 1 : Subsystem
  Comparator 10 : Subsystem
  Comparator 11 : Subsystem
  Comparator 12 : Subsystem
  Comparator 13 : Subsystem
  Comparator 14 : Subsystem
  Comparator 2 : Subsystem
  Comparator 3 : Subsystem
  Comparator 4 : Subsystem
  Comparator 5 : Subsystem
  Comparator 6 : Subsystem
  Comparator 7 : Subsystem
  Comparator 8 : Subsystem
  Comparator 9 : Subsystem
  Vref 1 : Constant  Value=-13/16
  Vref 10 : Constant  Value=5/16
  Vref 11 : Constant  Value=7/16
  Vref 12 : Constant  Value=9/16
  Vref 13 : Constant  Value=11/16
  Vref 14 : Constant  Value=13/16
  Vref 2 : Constant  Value=-11/16
  Vref 3 : Constant  Value=-9/16
  Vref 4 : Constant  Value=-7/16
  Vref 5 : Constant  Value=-5/16
  Vref 6 : Constant  Value=-3/16
  Vref 7 : Constant  Value=-1/16
  Vref 8 : Constant  Value=1/16
  Vref 9 : Constant  Value=3/16
  b1 : Outport
  b2 : Outport  Port=2
  b3 : Outport  Port=3
  b4 : Outport  Port=4
  b5 : Outport  Port=5
  b6 : Outport  Port=6
  b7 : Outport  Port=7
  b8 : Outport  Port=8
  b9 : Outport  Port=9
  b10 : Outport  Port=10
  b11 : Outport  Port=11
  b12 : Outport  Port=12
  b13 : Outport  Port=13
  b14 : Outport  Port=14
  wires:
  Vin/1 -> Comparator 1/1(Vin), Comparator 2/1(Vin), Comparator 3/1(Vin), Comparator 4/1(Vin), Comparator 5/1(Vin), Comparator 6/1(Vin), Comparator 7/1(Vin), Comparator 8/1(Vin), Comparator 9/1(Vin), Comparator 10/1(Vin), Comparator 11/1(Vin), Comparator 12/1(Vin), Comparator 13/1(Vin), Comparator 14/1(Vin)
  Vref 1/1 -> Comparator 1/2(Vref)
  Vref 2/1 -> Comparator 2/2(Vref)
  Vref 14/1 -> Comparator 14/2(Vref)
  Vref 4/1 -> Comparator 4/2(Vref)
  Vref 5/1 -> Comparator 5/2(Vref)
  Vref 12/1 -> Comparator 12/2(Vref)
  Comparator 9/1(b9) -> b9/1
  Vref 9/1 -> Comparator 9/2(Vref)
  Comparator 5/1(b5) -> b5/1
  Vref 13/1 -> Comparator 13/2(Vref)
  Vref 6/1 -> Comparator 6/2(Vref)
  Vref 7/1 -> Comparator 7/2(Vref)
  Comparator 2/1(b2) -> b2/1
  Vref 3/1 -> Comparator 3/2(Vref)
  Vref 10/1 -> Comparator 10/2(Vref)
  Comparator 11/1(b11) -> b11/1
  Vref 8/1 -> Comparator 8/2(Vref)
  Vref 11/1 -> Comparator 11/2(Vref)
  Comparator 12/1(b12) -> b12/1
  Comparator 13/1(b13) -> b13/1
  Comparator 10/1(b10) -> b10/1
  Comparator 1/1(b1) -> b1/1
  Comparator 4/1(b4) -> b4/1
  Comparator 8/1(b8) -> b8/1
  Comparator 7/1(b7) -> b7/1
  Comparator 14/1(b14) -> b14/1
  Comparator 3/1(b3) -> b3/1
  Comparator 6/1(b6) -> b6/1

== system pipeline_13bit/13_bit/Subsystem/stage_3p5_bit/Sub DAC ==
  b1 : Inport
  b2 : Inport  Port=2
  b3 : Inport  Port=3
  b4 : Inport  Port=4
  b5 : Inport  Port=5
  b6 : Inport  Port=6
  b7 : Inport  Port=7
  b8 : Inport  Port=8
  b9 : Inport  Port=9
  b10 : Inport  Port=10
  b11 : Inport  Port=11
  b12 : Inport  Port=12
  b13 : Inport  Port=13
  b14 : Inport  Port=14
  Constant : Constant  Value=14
  Gain : Gain  Gain=2
  Gain1 : Gain  Gain=0.5
  Sum : Sum  Inputs=++++++++++++++
  Sum1 : Sum  Inputs=|+-
  Vdac : Outport
  wires:
  Sum/1 -> Gain/1
  Gain/1 -> Sum1/1
  Constant/1 -> Sum1/2
  Sum1/1 -> Gain1/1
  Gain1/1 -> Vdac/1
  b1/1 -> Sum/1
  b2/1 -> Sum/2
  b3/1 -> Sum/3
  b4/1 -> Sum/4
  b5/1 -> Sum/5
  b6/1 -> Sum/6
  b7/1 -> Sum/7
  b8/1 -> Sum/8
  b9/1 -> Sum/9
  b10/1 -> Sum/10
  b11/1 -> Sum/11
  b12/1 -> Sum/12
  b13/1 -> Sum/13
  b14/1 -> Sum/14

== system pipeline_13bit/13_bit/Subsystem/stage_3p5_bit/Subsystem1 ==
  IN : Inport
  Clock Jitter : Subsystem  Description=Jitter
  Gain : Gain
  Saturation : Saturate  UpperLimit=1000  LowerLimit=-1
  Zero-Order Hold1 : ZeroOrderHold  SampleTime=ts
  S/H : Outport
  wires:
  Zero-Order Hold1/1 -> S/H/1
  Saturation/1 -> Zero-Order Hold1/1
  IN/1 -> Clock Jitter/1(IN)
  Clock Jitter/1(Clock) -> Gain/1
  Gain/1 -> Saturation/1

== system pipeline_13bit/SHA_less_13_bit/Subsystem/stage_1p5_bit1/Comparator 1 ==
  Vin : Inport
  Vref : Inport  Port=2
  Output 1 or 0 : Relay  OnSwitchValue=0  OffSwitchValue=0
  Sum : Sum  Inputs=|+-
  Out : Outport
  wires:
  Sum/1 -> Output 1 or 0/1
  Vin/1 -> Sum/1
  Output 1 or 0/1 -> Out/1
  Vref/1 -> Sum/2

== system pipeline_13bit/SHA_less_13_bit/Subsystem/stage_1p5_bit1/Comparator 2 ==
  Vin : Inport
  Vref : Inport  Port=2
  Output 1 or 0 : Relay  OnSwitchValue=0  OffSwitchValue=0
  Sum : Sum  Inputs=|+-
  Out : Outport
  wires:
  Sum/1 -> Output 1 or 0/1
  Vin/1 -> Sum/1
  Output 1 or 0/1 -> Out/1
  Vref/1 -> Sum/2

== system pipeline_13bit/SHA_less_13_bit/Subsystem/stage_1p5_bit1/Encoder ==
  b1 : Inport
  b2 : Inport  Port=2
  " " : DataTypeConversion  OutDataTypeStr=double  SaturateOnIntegerOverflow=off  RndMeth=Floor
  NOR : Logic  Operator=NOR  AllPortsSameDT=off  OutDataTypeStr=boolean
  NOT : Logic  Operator=NOT  AllPortsSameDT=off  OutDataTypeStr=boolean
  D0 : Outport
  D1 : Outport  Port=2
  wires:
  b2/1 -> NOR/2, D1/1
  NOR/1 -> " "/1
  " "/1 -> D0/1
  NOT/1 -> NOR/1
  b1/1 -> NOT/1

== system pipeline_13bit/SHA_less_13_bit/Subsystem/stage_1p5_bit1/Sub DAC ==
  b1 : Inport
  b2 : Inport  Port=2
  NOT : Logic  Operator=NOT  AllPortsSameDT=off  OutDataTypeStr=boolean
  Subtract : Sum  Inputs=-+
  Vdac : Outport
  wires:
  b2/1 -> Subtract/2
  b1/1 -> NOT/1
  Subtract/1 -> Vdac/1
  NOT/1 -> Subtract/1

== system pipeline_13bit/SHA_less_13_bit/Subsystem/stage_1p5_bit1/Subsystem1 ==
  IN : Inport
  Clock Jitter : Subsystem  Description=Jitter
  Gain : Gain
  Saturation : Saturate  UpperLimit=1000  LowerLimit=-1
  Zero-Order Hold1 : ZeroOrderHold  SampleTime=ts
  S/H : Outport
  wires:
  Zero-Order Hold1/1 -> S/H/1
  Saturation/1 -> Zero-Order Hold1/1
  IN/1 -> Clock Jitter/1(IN)
  Clock Jitter/1(Clock) -> Gain/1
  Gain/1 -> Saturation/1

== system pipeline_13bit/SHA_less_13_bit/Subsystem/stage_1p5_bit2/Comparator 1 ==
  Vin : Inport
  Vref : Inport  Port=2
  Output 1 or 0 : Relay  OnSwitchValue=0  OffSwitchValue=0
  Sum : Sum  Inputs=|+-
  Out : Outport
  wires:
  Sum/1 -> Output 1 or 0/1
  Vin/1 -> Sum/1
  Output 1 or 0/1 -> Out/1
  Vref/1 -> Sum/2

== system pipeline_13bit/SHA_less_13_bit/Subsystem/stage_1p5_bit2/Comparator 2 ==
  Vin : Inport
  Vref : Inport  Port=2
  Output 1 or 0 : Relay  OnSwitchValue=0  OffSwitchValue=0
  Sum : Sum  Inputs=|+-
  Out : Outport
  wires:
  Sum/1 -> Output 1 or 0/1
  Vin/1 -> Sum/1
  Output 1 or 0/1 -> Out/1
  Vref/1 -> Sum/2

== system pipeline_13bit/SHA_less_13_bit/Subsystem/stage_1p5_bit2/Encoder ==
  b1 : Inport
  b2 : Inport  Port=2
  " " : DataTypeConversion  OutDataTypeStr=double  SaturateOnIntegerOverflow=off  RndMeth=Floor
  NOR : Logic  Operator=NOR  AllPortsSameDT=off  OutDataTypeStr=boolean
  NOT : Logic  Operator=NOT  AllPortsSameDT=off  OutDataTypeStr=boolean
  D0 : Outport
  D1 : Outport  Port=2
  wires:
  b2/1 -> NOR/2, D1/1
  NOR/1 -> " "/1
  " "/1 -> D0/1
  NOT/1 -> NOR/1
  b1/1 -> NOT/1

== system pipeline_13bit/SHA_less_13_bit/Subsystem/stage_1p5_bit2/Sub DAC ==
  b1 : Inport
  b2 : Inport  Port=2
  NOT : Logic  Operator=NOT  AllPortsSameDT=off  OutDataTypeStr=boolean
  Subtract : Sum  Inputs=-+
  Vdac : Outport
  wires:
  b2/1 -> Subtract/2
  b1/1 -> NOT/1
  Subtract/1 -> Vdac/1
  NOT/1 -> Subtract/1

== system pipeline_13bit/SHA_less_13_bit/Subsystem/stage_1p5_bit2/Subsystem1 ==
  IN : Inport
  Clock Jitter : Subsystem  Description=Jitter
  Gain : Gain
  Saturation : Saturate  UpperLimit=1000  LowerLimit=-1
  Zero-Order Hold1 : ZeroOrderHold  SampleTime=ts
  S/H : Outport
  wires:
  Zero-Order Hold1/1 -> S/H/1
  Saturation/1 -> Zero-Order Hold1/1
  IN/1 -> Clock Jitter/1(IN)
  Clock Jitter/1(Clock) -> Gain/1
  Gain/1 -> Saturation/1

== system pipeline_13bit/SHA_less_13_bit/Subsystem/stage_1p5_bit4/Comparator 1 ==
  Vin : Inport
  Vref : Inport  Port=2
  Output 1 or 0 : Relay  OnSwitchValue=0  OffSwitchValue=0
  Sum : Sum  Inputs=|+-
  Out : Outport
  wires:
  Sum/1 -> Output 1 or 0/1
  Vin/1 -> Sum/1
  Output 1 or 0/1 -> Out/1
  Vref/1 -> Sum/2

== system pipeline_13bit/SHA_less_13_bit/Subsystem/stage_1p5_bit4/Comparator 2 ==
  Vin : Inport
  Vref : Inport  Port=2
  Output 1 or 0 : Relay  OnSwitchValue=0  OffSwitchValue=0
  Sum : Sum  Inputs=|+-
  Out : Outport
  wires:
  Sum/1 -> Output 1 or 0/1
  Vin/1 -> Sum/1
  Output 1 or 0/1 -> Out/1
  Vref/1 -> Sum/2

== system pipeline_13bit/SHA_less_13_bit/Subsystem/stage_1p5_bit4/Encoder ==
  b1 : Inport
  b2 : Inport  Port=2
  " " : DataTypeConversion  OutDataTypeStr=double  SaturateOnIntegerOverflow=off  RndMeth=Floor
  NOR : Logic  Operator=NOR  AllPortsSameDT=off  OutDataTypeStr=boolean
  NOT : Logic  Operator=NOT  AllPortsSameDT=off  OutDataTypeStr=boolean
  D0 : Outport
  D1 : Outport  Port=2
  wires:
  b2/1 -> NOR/2, D1/1
  NOR/1 -> " "/1
  " "/1 -> D0/1
  NOT/1 -> NOR/1
  b1/1 -> NOT/1

== system pipeline_13bit/SHA_less_13_bit/Subsystem/stage_1p5_bit4/Sub DAC ==
  b1 : Inport
  b2 : Inport  Port=2
  NOT : Logic  Operator=NOT  AllPortsSameDT=off  OutDataTypeStr=boolean
  Subtract : Sum  Inputs=-+
  Vdac : Outport
  wires:
  b2/1 -> Subtract/2
  b1/1 -> NOT/1
  Subtract/1 -> Vdac/1
  NOT/1 -> Subtract/1

== system pipeline_13bit/SHA_less_13_bit/Subsystem/stage_1p5_bit4/Subsystem1 ==
  IN : Inport
  Clock Jitter : Subsystem  Description=Jitter
  Gain : Gain
  Saturation : Saturate  UpperLimit=1000  LowerLimit=-1
  Zero-Order Hold1 : ZeroOrderHold  SampleTime=ts
  S/H : Outport
  wires:
  Zero-Order Hold1/1 -> S/H/1
  Saturation/1 -> Zero-Order Hold1/1
  IN/1 -> Clock Jitter/1(IN)
  Clock Jitter/1(Clock) -> Gain/1
  Gain/1 -> Saturation/1

== system pipeline_13bit/SHA_less_13_bit/Subsystem/stage_1p5_bit5/Comparator 1 ==
  Vin : Inport
  Vref : Inport  Port=2
  Output 1 or 0 : Relay  OnSwitchValue=0  OffSwitchValue=0
  Sum : Sum  Inputs=|+-
  Out : Outport
  wires:
  Sum/1 -> Output 1 or 0/1
  Vin/1 -> Sum/1
  Output 1 or 0/1 -> Out/1
  Vref/1 -> Sum/2

== system pipeline_13bit/SHA_less_13_bit/Subsystem/stage_1p5_bit5/Comparator 2 ==
  Vin : Inport
  Vref : Inport  Port=2
  Output 1 or 0 : Relay  OnSwitchValue=0  OffSwitchValue=0
  Sum : Sum  Inputs=|+-
  Out : Outport
  wires:
  Sum/1 -> Output 1 or 0/1
  Vin/1 -> Sum/1
  Output 1 or 0/1 -> Out/1
  Vref/1 -> Sum/2

== system pipeline_13bit/SHA_less_13_bit/Subsystem/stage_1p5_bit5/Encoder ==
  b1 : Inport
  b2 : Inport  Port=2
  " " : DataTypeConversion  OutDataTypeStr=double  SaturateOnIntegerOverflow=off  RndMeth=Floor
  NOR : Logic  Operator=NOR  AllPortsSameDT=off  OutDataTypeStr=boolean
  NOT : Logic  Operator=NOT  AllPortsSameDT=off  OutDataTypeStr=boolean
  D0 : Outport
  D1 : Outport  Port=2
  wires:
  b2/1 -> NOR/2, D1/1
  NOR/1 -> " "/1
  " "/1 -> D0/1
  NOT/1 -> NOR/1
  b1/1 -> NOT/1

== system pipeline_13bit/SHA_less_13_bit/Subsystem/stage_1p5_bit5/Sub DAC ==
  b1 : Inport
  b2 : Inport  Port=2
  NOT : Logic  Operator=NOT  AllPortsSameDT=off  OutDataTypeStr=boolean
  Subtract : Sum  Inputs=-+
  Vdac : Outport
  wires:
  b2/1 -> Subtract/2
  b1/1 -> NOT/1
  Subtract/1 -> Vdac/1
  NOT/1 -> Subtract/1

== system pipeline_13bit/SHA_less_13_bit/Subsystem/stage_1p5_bit5/Subsystem1 ==
  IN : Inport
  Clock Jitter : Subsystem  Description=Jitter
  Gain : Gain
  Saturation : Saturate  UpperLimit=1000  LowerLimit=-1
  Zero-Order Hold1 : ZeroOrderHold  SampleTime=ts
  S/H : Outport
  wires:
  Zero-Order Hold1/1 -> S/H/1
  Saturation/1 -> Zero-Order Hold1/1
  IN/1 -> Clock Jitter/1(IN)
  Clock Jitter/1(Clock) -> Gain/1
  Gain/1 -> Saturation/1

== system pipeline_13bit/SHA_less_13_bit/Subsystem/stage_1p5_bit6/Comparator 1 ==
  Vin : Inport
  Vref : Inport  Port=2
  Output 1 or 0 : Relay  OnSwitchValue=0  OffSwitchValue=0
  Sum : Sum  Inputs=|+-
  Out : Outport
  wires:
  Sum/1 -> Output 1 or 0/1
  Vin/1 -> Sum/1
  Output 1 or 0/1 -> Out/1
  Vref/1 -> Sum/2

== system pipeline_13bit/SHA_less_13_bit/Subsystem/stage_1p5_bit6/Comparator 2 ==
  Vin : Inport
  Vref : Inport  Port=2
  Output 1 or 0 : Relay  OnSwitchValue=0  OffSwitchValue=0
  Sum : Sum  Inputs=|+-
  Out : Outport
  wires:
  Sum/1 -> Output 1 or 0/1
  Vin/1 -> Sum/1
  Output 1 or 0/1 -> Out/1
  Vref/1 -> Sum/2

== system pipeline_13bit/SHA_less_13_bit/Subsystem/stage_1p5_bit6/Encoder ==
  b1 : Inport
  b2 : Inport  Port=2
  " " : DataTypeConversion  OutDataTypeStr=double  SaturateOnIntegerOverflow=off  RndMeth=Floor
  NOR : Logic  Operator=NOR  AllPortsSameDT=off  OutDataTypeStr=boolean
  NOT : Logic  Operator=NOT  AllPortsSameDT=off  OutDataTypeStr=boolean
  D0 : Outport
  D1 : Outport  Port=2
  wires:
  b2/1 -> NOR/2, D1/1
  NOR/1 -> " "/1
  " "/1 -> D0/1
  NOT/1 -> NOR/1
  b1/1 -> NOT/1

== system pipeline_13bit/SHA_less_13_bit/Subsystem/stage_1p5_bit6/Sub DAC ==
  b1 : Inport
  b2 : Inport  Port=2
  NOT : Logic  Operator=NOT  AllPortsSameDT=off  OutDataTypeStr=boolean
  Subtract : Sum  Inputs=-+
  Vdac : Outport
  wires:
  b2/1 -> Subtract/2
  b1/1 -> NOT/1
  Subtract/1 -> Vdac/1
  NOT/1 -> Subtract/1

== system pipeline_13bit/SHA_less_13_bit/Subsystem/stage_1p5_bit6/Subsystem1 ==
  IN : Inport
  Clock Jitter : Subsystem  Description=Jitter
  Gain : Gain
  Saturation : Saturate  UpperLimit=1000  LowerLimit=-1
  Zero-Order Hold1 : ZeroOrderHold  SampleTime=ts
  S/H : Outport
  wires:
  Zero-Order Hold1/1 -> S/H/1
  Saturation/1 -> Zero-Order Hold1/1
  IN/1 -> Clock Jitter/1(IN)
  Clock Jitter/1(Clock) -> Gain/1
  Gain/1 -> Saturation/1

== system pipeline_13bit/SHA_less_13_bit/Subsystem/stage_1p5_bit7/Comparator 1 ==
  Vin : Inport
  Vref : Inport  Port=2
  Output 1 or 0 : Relay  OnSwitchValue=0  OffSwitchValue=0
  Sum : Sum  Inputs=|+-
  Out : Outport
  wires:
  Sum/1 -> Output 1 or 0/1
  Vin/1 -> Sum/1
  Output 1 or 0/1 -> Out/1
  Vref/1 -> Sum/2
